simulink model "identificacion2"  (R2018a)
settings: Solver=VariableStepAuto  StartTime=0.0  StopTime=300  RelTol=1e-3
undefined symbols (not defined in the file or in its folder): tf1, tf2
libraries: instrumentlib x1
settings Model: Creator=carma  LastModifiedBy=carma

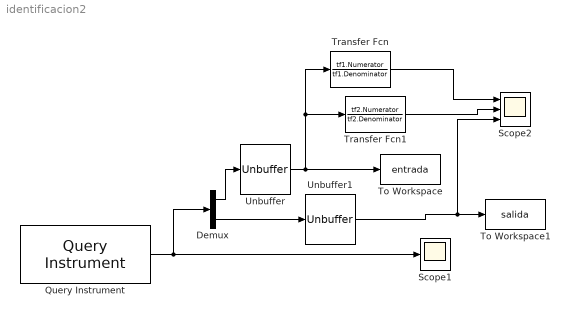
== system identificacion2 ==
  Demux : Demux  Outputs=2
  Query Instrument : instrumentlib/Query Instrument  sampleTime=1  isWorkspaceObject=off  timeout=10  inputBufferSize=512  protocol=Serial  serialPort=COM1  baudRate=115200  gpibVendor=Keysight Technologies  boardIndex=0  primaryAddress=1  secondaryAddress=0  visaVendor=Keysight  visaSerialPort=0  chassisIndex=0  logicalAddress=0  tcpRemoteHost='127.0.0.1'  tcpRemotePort=4500  udpRemoteHost='127.0.0.1'  udpRemotePort=9090  visaTCPBoardIndex=0  visaTCPRemoteHost='127.0.0.1'  usbBoardIndex=0  usbManufID=0  usbModelCode=0  usbSerialNumber=0  initAction=None  initCommand='DATA:SOURCE CH1'  initFunction=get  queryCommand=''  responseFormat=ASCII  asciiFormatting='%f,%f\n'  precision=8-bit integer  byteOrder=Little endian  valuesToRead=1  removeBytes=on  afterOutputAction=Repeat query for new data  enableFrames=on  frameSize=2
      settings: SourceProductName=Instrument Control Toolbox  SourceProductBaseCode=IC
  Scope1 : Scope
  Scope2 : Scope  NumInputPorts=3
  To Workspace : ToWorkspace  VariableName=entrada  SampleTime=1
      settings: Save2DSignal=2-D array (concatenate along first dimension)
  To Workspace1 : ToWorkspace  VariableName=salida  SampleTime=1
      settings: Save2DSignal=2-D array (concatenate along first dimension)
  Transfer Fcn : TransferFcn  Numerator=tf1.Numerator  Denominator=tf1.Denominator
  Transfer Fcn1 : TransferFcn  Numerator=tf2.Numerator  Denominator=tf2.Denominator
  Unbuffer : Unbuffer
  Unbuffer1 : Unbuffer
  wires:
  Query Instrument/1 -> Demux/1, Scope1/1
  Demux/1 -> Unbuffer/1
  Demux/2 -> Unbuffer1/1
  Unbuffer/1 -> Transfer Fcn1/1, Transfer Fcn/1, To Workspace/1
  Unbuffer1/1 -> Scope2/3, To Workspace1/1
  Transfer Fcn/1 -> Scope2/1
  Transfer Fcn1/1 -> Scope2/2
